simulink model "Erweiterung2"  (R2015a)
settings: Solver=ode45  StartTime=0.0  StopTime=10.0  RelTol=1e-3
InitFcn:
  | Sollwert_Zusatz
undefined symbols (not defined in the file or in its folder): C1, C2, L1, L2, R1, R2, RL
settings Model: Creator=cds-lue-1  LastModifiedBy=cds-lue-1

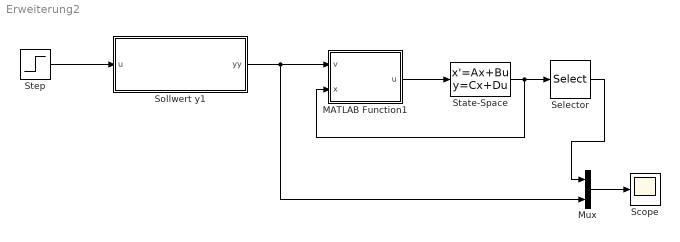
== system Erweiterung2 ==
  MATLAB Function1 : MATLAB Function  TreatAsAtomicUnit=on
  Mux : Mux  Inputs=2
  Scope : Scope
  Selector : Selector  InputPortWidth=4  Indices=[3]
  Sollwert y1 : MATLAB Function  TreatAsAtomicUnit=on  SystemSampleTime=0.001
  State-Space : StateSpace  A=[-R1 / L1 -0.1e1 / L1 0 0; 0.1e1 / C1 0 -0.1e1 / C1 0; 0 0.1e1 / L2 -R2 / L2 -0.1e1 / L2; 0 0 0.1e1 / C2 -0.1e1 / C2 / RL;]  B=[0.1e1 / L1; 0; 0; 0;]  C=eye(4)  D=zeros(4,1)  X0=0
  Step : Step  SampleTime=0
  wires:
  Step/1 -> Sollwert y1/1(u)
  State-Space/1 -> Selector/1, MATLAB Function1/2(x)
  Sollwert y1/1(yy) -> MATLAB Function1/1(v), Mux/2
  Mux/1 -> Scope/1
  MATLAB Function1/1(u) -> State-Space/1
  Selector/1 -> Mux/1

== matlab function Erweiterung2/Sollwert y1 ==
  settings: updateMethod=DISCRETE  sampleTime=parSollwertfilter.Ta
  data: u input; yy output; parSollwertfilter parameter
function yy  = sollwertfilter(u,  parSollwertfilter)
persistent x;
% Anfangswert abziehen

a=parSollwertfilter.a;
b=parSollwertfilter.b;
c=parSollwertfilter.c;
d=parSollwertfilter.d;

if(isempty(x))
     x=[0;0;0;0];
end

yt=c*x+d*u;

yy = yt;

x=a*x+b*u;

== matlab function Erweiterung2/MATLAB Function1 ==
  data: u output; v input; x input
function u  = fcn(v,x)
%#codegen
L1=0.3;
L2=0.1;
C1=0.1;
C2=0.2;
R1=0.5;
R2=0.1;
RL=500;

if(isempty(x))
     x=[0;0;0;0];
end


A = [-R1 / L1 -0.1e1 / L1 0 0; 0.1e1 / C1 0 -0.1e1 / C1 0; 0 0.1e1 / L2 -R2 / L2 -0.1e1 / L2; 0 0 0.1e1 / C2 -0.1e1 / C2 / RL];
b = [0.1e1 / L1; 0; 0; 0];
c = [0; 0; 1; 0];

u=(-c'*A*A*A*x+v)/(c'*A*A*b);
